simulink model "ModelloSimulink[1976917]"  (R2021a)
settings: Solver=VariableStepAuto  StartTime=0.0  StopTime=2  RelTol=1e-3
values from neighbouring files (symbols this model uses):
  A = m*e*(omega^2)    [DatiIngressoSimulazione.m]
  c1 = 1.5*c    [DatiIngressoSimulazione.m]
  k1 = k*1.5    [DatiIngressoSimulazione.m]
  M = input(prompt)    [DatiIngressoSimulazione.m]
  omega = 0.14072*rpm    [DatiIngressoSimulazione.m]
settings Model: Creator=Franco Del Mastro  LastModifiedBy=Franco Del Mastro

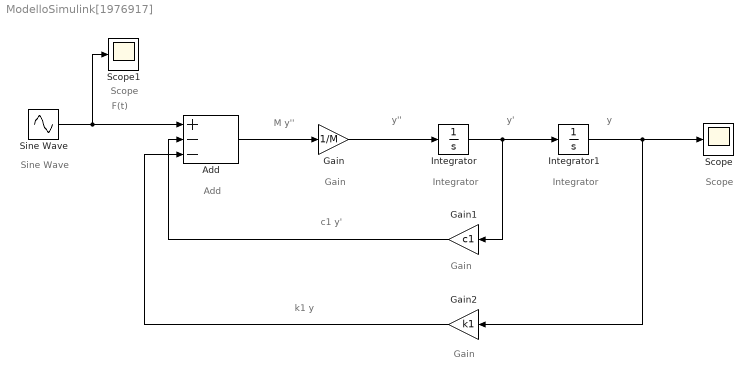
== system ModelloSimulink[1976917] ==
  note: Integrator
  note: c1 y'
  note: k1 y
  note: M y''
  note: F(t)
  note: y'
  note: y
  note: y''
  note: Integrator
  note: Gain
  note: Gain
  note: Gain
  note: Scope
  note: Add
  note: Sine Wave
  note: Scope
  Add : Sum  Inputs=+--
  Gain : Gain  Gain=1/M
  Gain1 : Gain  Gain=c1
  Gain2 : Gain  Gain=k1
  Integrator : Integrator
  Integrator1 : Integrator
  Scope : Scope
  Scope1 : Scope
  Sine Wave : Sin  Amplitude=A  Frequency=omega  SampleTime=0
  wires:
  Add/1 -> Gain/1
  Gain/1 -> Integrator/1
  Integrator/1 -> Gain1/1, Integrator1/1
  Gain1/1 -> Add/2
  Gain2/1 -> Add/3
  Integrator1/1 -> Gain2/1, Scope/1
  Sine Wave/1 -> Scope1/1, Add/1
